simulink model "Problem8"  (R2020b)
settings: Solver=VariableStepAuto  StartTime=0.0  StopTime=10.0  RelTol=1e-3
settings Model: Creator=amolg  LastModifiedBy=amolg

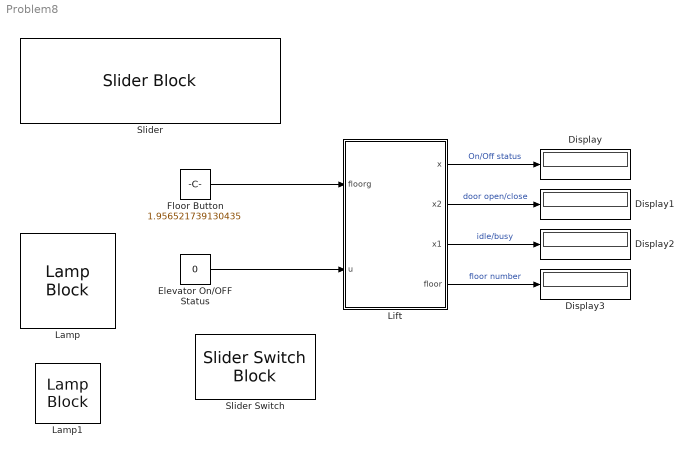
== system Problem8 ==
  Display{,1..3} (4 alike) : Display
  Elevator On/OFF Status : Constant  Value=0
  Floor Button : Constant  Value=1.956521739130435
  Lamp : LampBlock
  Lamp1 : LampBlock
  Lift : Stateflow chart  TreatAsAtomicUnit=on
  Slider : SliderBlock  ScaleMax=5  TickInterval=1
  Slider Switch : SliderSwitchBlock
      settings: Values={{'Off', 'On'}, [0 1]}
  wires:
  Lift/1(x) -> Display/1  "On/Off status"
  Lift/2(x2) -> Display1/1  "door open/close"
  Lift/4(floor) -> Display3/1  "floor number"
  Floor Button/1 -> Lift/1(floorg)
  Elevator On/OFF Status/1 -> Lift/2(u)
  Lift/3(x1) -> Display2/1  "idle/busy"

== stateflow chart Problem8/Lift ==
  state Elevator_on
    entry: x=1;
    note: [floorb<floor]{y1= 1 }
    state DOWN
      entry:
      floor=floor-1;
    state Delay1
      entry:
      floor=floor-1;
    state Idle_state
      entry: x1=0;
    state UP
      entry:
      floor=floor+1;
    state Delay
      entry:
      floor=floor+1;
    state Door_open1
      entry:
      x2=1;
    state Door_close1
      entry:
      x2=0;
    state Door_open
      entry:
      x2=1;
    state Door_close
      entry:
      x2=0;
    (default) -> Idle_state
    DOWN -> Delay1 [order 1] : [floorg<floor]
    Idle_state -> DOWN [order 2]
    Delay1 -> DOWN [order 1] : [floorg<floor]
    Idle_state -> UP [order 1] : [floorg>floor]{x1=1}
    DOWN -> Door_open1 [order 2] : [floorg==floor]
    Delay1 -> Door_open1 [order 2] : [floor==floorg]
    Delay -> UP [order 1] : [floorg>floor]
    UP -> Delay [order 1] : [floorg>floor]
    UP -> Door_open [order 2] : [floorg==floor]
    Delay -> Door_open [order 2] : [floor==floorg]
    Door_open1 -> Door_close1 : [after(5,sec)]
    Door_open -> Door_close : [after(5,sec)]
  state Elevator_off
    entry: x=0;
  (default) -> Elevator_on
  Elevator_on -> Elevator_off : [u==0]
  Elevator_off -> Elevator_on : [u==1]
  data: floorg input [0..5]; u input; x output [0..1]; x2 output [0..1]; x1 output [0..1]; floor output [0..5] =0
